simulink model "DCM_Sensing"  (R2019a)
settings: Solver=ode5  StartTime=0.0  StopTime=t_end  FixedStep=dt  RelTol=1e-3  EnableMultiTasking=on
values from neighbouring files (symbols this model uses):
  dt = 1e-5    (= 1e-05)    [Experiment_1_DCM_Parameter.m]
  dt_omega = 5e-4    (= 0.0005)    [Experiment_1_DCM_Parameter.m]
  EncoderLines = 4096    [Experiment_1_DCM_Parameter.m]
  I_AN = 1    [Experiment_1_DCM_Parameter.m]
  I_EN = 0.1    [Experiment_1_DCM_Parameter.m]
  n_Igain = 0.075    [Experiment_1_DCM_Parameter.m]
  n_Imax = 0.15    [Experiment_1_DCM_Parameter.m]
  n_Imin = -n_Imax    (= -0.15)    [Experiment_1_DCM_Parameter.m]
  T_CON = 0    [Experiment_1_DCM_Parameter.m]
  V_CON = 0    [Experiment_1_DCM_Parameter.m]
libraries: simulink x3
settings Model: Creator=BinLi  LastModifiedBy=Praktikum
settings DataIOCC: LimitDataPoints=on  SaveFormat=Array  SignalLoggingSaveFormat=ModelDataLogs  ReturnWorkspaceOutputs=off
settings OptimizationCC: ExpressionDepthLimit=2147483647  LifeSpan=inf
settings DebuggingCC: UnderspecifiedInitializationDetection=Classic  MergeDetectMultiDrivingBlocksExec=none  SolverPrmCheckMsg=warning  FcnCallInpInsideContextMsg=warning  StateNameClashWarn=warning  SFUnexpectedBacktrackingDiag=warning  SFNoUnconditionalDefaultTransitionDiag=warning  SFExecutionAtInitializationDiag=none  ArithmeticOperatorsInVariantConditions=warning
settings HardwareCC: ProdBitPerPointer=32  ProdBitPerSizeT=32  ProdBitPerPtrDiffT=32  ProdLargestAtomicFloat=None  ProdIntDivRoundTo=Undefined  ProdEndianess=Unspecified  ProdWordSize=32  ProdHWDeviceType=32-bit Generic
settings ModelReferenceCC: PropagateSignalLabelsOutOfModel=off
settings SFSimCC: SimUseLocalCustomCode=off
settings RTWCC: RTWUseLocalCustomCode=off
settings CodeAppCC: StateflowObjectComments=on
settings GRTTargetCC: TargetLangStandard=C89/C90 (ANSI)  CombineOutputUpdateFcns=off  GRTInterface=on
settings ConfigComp: CovMetricSettings=dw  CovSaveCumulativeToWorkspaceVar=on  CovSaveSingleToWorkspaceVar=on  CovExternalEMLEnable=off  CovSFcnEnable=off

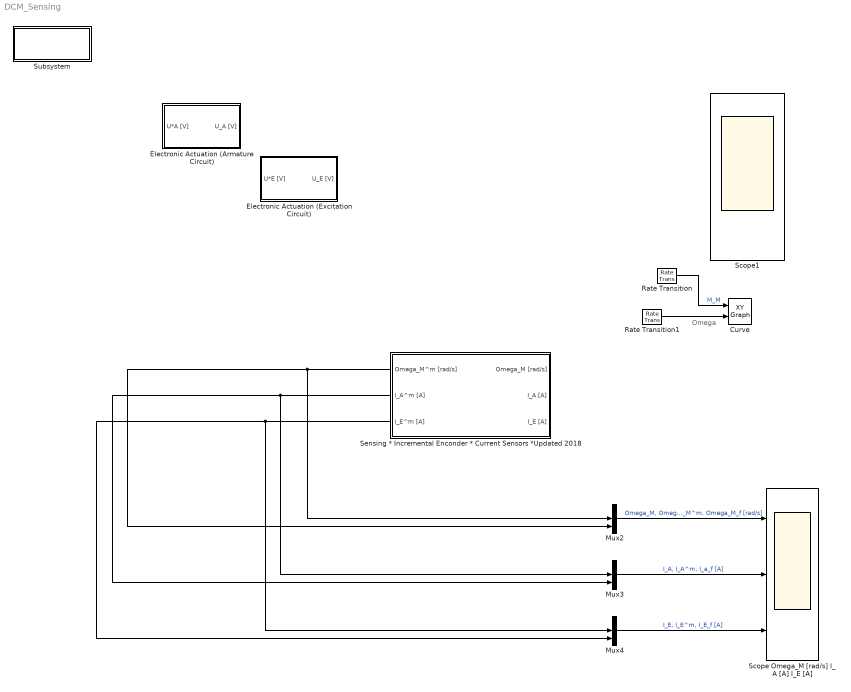
== system DCM_Sensing ==
  note: Omega
  Curve : simulink/Sinks/XY Graph  xmin=-1000  xmax=1200  ymin=-2000  ymax=2000  st=5e-3
  Electronic Actuation (Armature Circuit) : Subsystem
  Electronic Actuation (Excitation Circuit) : Subsystem
  Mux2 : Mux  Inputs=3
  Mux3 : Mux  Inputs=3
  Mux4 : Mux  Inputs=3
  Rate Transition : RateTransition
  Rate Transition1 : RateTransition
  Scope Omega_M [rad/s] I_A [A] I_E [A] : Scope  NumInputPorts=3
  Scope1 : Scope  NumInputPorts=6
  Sensing * Incremental Enconder * Current Sensors *Updated 2018 : Subsystem
  Subsystem : Subsystem
      settings: OpenFcn=Experiment_1_DCM_Parameter
      mask Display: disp('Initialize\n (doppelklicken)')
  wires:
  ? -> Scope1/1, Rate Transition1/1, Sensing * Incremental Enconder * Current Sensors *Updated 2018/1(Omega_M [rad/s]), Mux2/1  "Omega"
  ? -> Scope1/2, Sensing * Incremental Enconder * Current Sensors *Updated 2018/2(I_A [A]), Mux3/1  "I_A"
  ? -> Scope1/5, Sensing * Incremental Enconder * Current Sensors *Updated 2018/3(I_E [A]), Mux4/1  "I_E"
  ? -> Rate Transition/1, Scope1/6  "M_M"
  ? -> Scope1/3  "E_A"
  ? -> Scope1/4  "Psi_E"
  Rate Transition/1 -> Curve/1  "M_M"
  Rate Transition1/1 -> Curve/2
  Mux2/1 -> Scope Omega_M [rad/s] I_A [A] I_E [A]/1  "Omega_M, Omega_M^m, Omega_M_f [rad/s]"
  Mux3/1 -> Scope Omega_M [rad/s] I_A [A] I_E [A]/2  "I_A, I_A^m, I_a_f [A]"
  Mux4/1 -> Scope Omega_M [rad/s] I_A [A] I_E [A]/3  "I_E, I_E^m, I_E_f [A]"
  Sensing * Incremental Enconder * Current Sensors *Updated 2018/2(I_A^m [A]) -> Mux3/3, Mux3/2
  Sensing * Incremental Enconder * Current Sensors *Updated 2018/3(I_E^m [A]) -> Mux4/3, Mux4/2
  Sensing * Incremental Enconder * Current Sensors *Updated 2018/1(Omega_M^m [rad/s]) -> Mux2/3, Mux2/2

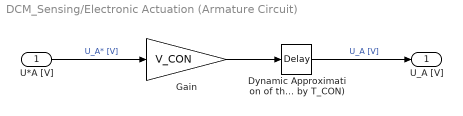
== system DCM_Sensing/Electronic Actuation (Armature Circuit) ==
  U*A [V] : Inport
  Dynamic Approximation of the 2-level-converter (Delay by T_CON) : TransportDelay  DelayTime=T_CON
  Gain : Gain  Gain=V_CON
  U_A [V] : Outport
  wires:
  Dynamic Approximation of the 2-level-converter (Delay by T_CON)/1 -> U_A [V]/1  "U_A [V]"
  U*A [V]/1 -> Gain/1  "U_A* [V]"
  Gain/1 -> Dynamic Approximation of the 2-level-converter (Delay by T_CON)/1

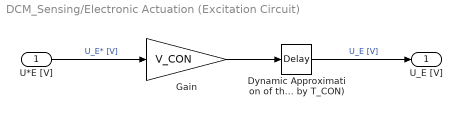
== system DCM_Sensing/Electronic Actuation (Excitation Circuit) ==
  U*E [V] : Inport
  Dynamic Approximation of the 2-level-converter (Delay by T_CON) : TransportDelay  DelayTime=T_CON
  Gain : Gain  Gain=V_CON
  U_E [V] : Outport
  wires:
  Gain/1 -> Dynamic Approximation of the 2-level-converter (Delay by T_CON)/1
  U*E [V]/1 -> Gain/1  "U_E* [V]"
  Dynamic Approximation of the 2-level-converter (Delay by T_CON)/1 -> U_E [V]/1  "U_E [V]"

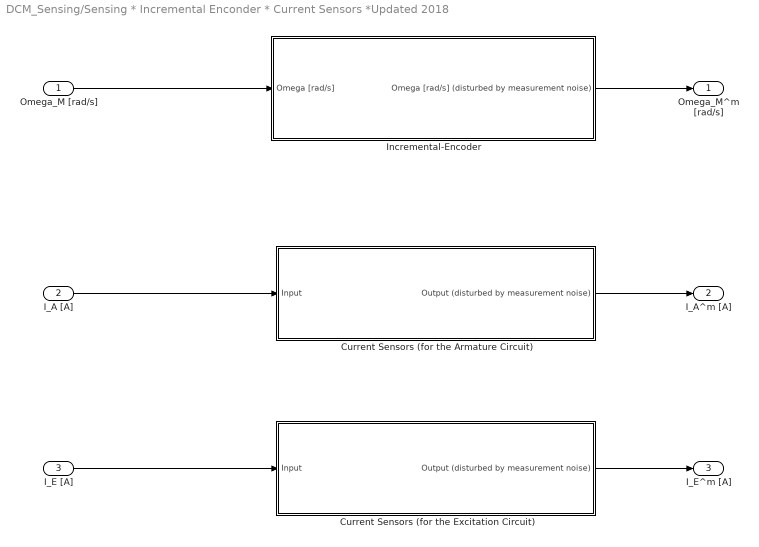
== system DCM_Sensing/Sensing * Incremental Enconder * Current Sensors *Updated 2018 ==
  Omega_M [rad/s] : Inport
  I_A [A] : Inport  Port=2
  I_E [A] : Inport  Port=3
  Current Sensors (for the Armature Circuit) : Subsystem  mask(Noise Generator){Noise_Power=0.1*dt, h_Noise=dt, V_Noise=n_Igain, Max_Noise=n_Imax*I_AN, Min_Noise=n_Imin*I_AN}
      mask prompts: Noise_Power "Noise Power (default: 0.1*h)"; h_Noise "Noise Sampling Time (default: h)"; V_Noise "Noise Gain (Amplification)"; Max_Noise "Maximal Noise Amplitude (Saturation)"; Min_Noise "Minimal Noise Amplitude (Saturation)"
      mask help:
      | This block generates sensor noise (band limited white noise) at a noise sampling time h_Noise [s, default: h] and with a noise power Noise_Power [1, default: 0.1*h], to produce normally distributed bandlimited white noise with a maximal amplitude around 1.
      | The noise amplitude can be amplified with a noise gain V_Noise [1] and saturated with the maximal and minimal noise amplitude selection.
      | With the flag "ENABLE_NOISE" (constant) the noise output can be activated or set to zero.
      mask Display:
      | fprintf('Noise Power: %1.3f [1]\n Noise Sampling Time: %1.3f [s] \n Noise Gain: %g [1] \n Saturation: [%g,%g]'...
      |    ,Noise_Power, h_Noise, V_Noise, Min_Noise, Max_Noise);
      | port_label('input',1,'I [A]');
      | port_label('output',1,'I^m [A]');
  "Current Sensors (for the Excitation Circuit) " : Subsystem  mask(Noise Generator){Noise_Power=0.1*dt, h_Noise=dt, V_Noise=n_Igain, Max_Noise=n_Imax*I_EN, Min_Noise=n_Imin*I_EN}
      mask prompts: Noise_Power "Noise Power (default: 0.1*h)"; h_Noise "Noise Sampling Time (default: h)"; V_Noise "Noise Gain (Amplification)"; Max_Noise "Maximal Noise Amplitude (Saturation)"; Min_Noise "Minimal Noise Amplitude (Saturation)"
      mask help:
      | This block generates sensor noise (band limited white noise) at a noise sampling time h_Noise [s, default: h] and with a noise power Noise_Power [1, default: 0.1*h], to produce normally distributed bandlimited white noise with a maximal amplitude around 1.
      | The noise amplitude can be amplified with a noise gain V_Noise [1] and saturated with the maximal and minimal noise amplitude selection.
      | With the flag "ENABLE_NOISE" (constant) the noise output can be activated or set to zero.
      mask Display:
      | fprintf('Noise Power: %1.3f [1]\n Noise Sampling Time: %1.3f [s] \n Noise Gain: %g [1] \n Saturation: [%g,%g]'...
      |    ,Noise_Power, h_Noise, V_Noise, Min_Noise, Max_Noise);
      | port_label('input',1,'I [A]');
      | port_label('output',1,'I^m [A]');
  Incremental-Encoder : Subsystem  mask(Noise Generator){enc_lines=EncoderLines}
      mask prompts: enc_lines "Encoder Lines"
      mask help:
      | This block generates sensor noise (band limited white noise) at a noise sampling time h_Noise [s, default: h] and with a noise power Noise_Power [1, default: 0.1*h], to produce normally distributed bandlimited white noise with a maximal amplitude around 1.
      | The noise amplitude can be amplified with a noise gain V_Noise [1] and saturated with the maximal and minimal noise amplitude selection.
      | With the flag "ENABLE_NOISE" (constant) the noise output can be activated or set to zero.
      mask Display:
      | fprintf('Encoder Lines %g [1]',enc_lines);
      | port_label('input',1,'Omega [rad/s]');
      | port_label('output',1,'Omega^m [rad/s]');
  Omega_M^m [rad/s] : Outport  InitialOutput=0
  I_A^m [A] : Outport  Port=2  InitialOutput=0
  I_E^m [A] : Outport  Port=3  InitialOutput=0
  wires:
  Omega_M [rad/s]/1 -> Incremental-Encoder/1(Omega [rad/s])
  I_A [A]/1 -> Current Sensors (for the Armature Circuit)/1(Input)
  I_E [A]/1 -> "Current Sensors (for the Excitation Circuit) "/1(Input)
  "Current Sensors (for the Excitation Circuit) "/1(Output (disturbed by measurement noise)) -> I_E^m [A]/1
  Current Sensors (for the Armature Circuit)/1(Output (disturbed by measurement noise)) -> I_A^m [A]/1
  Incremental-Encoder/1(Omega [rad/s] (disturbed by measurement noise)) -> Omega_M^m [rad/s]/1

== system DCM_Sensing/Subsystem ==

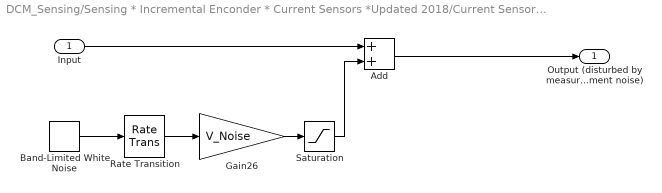
== system DCM_Sensing/Sensing * Incremental Enconder * Current Sensors *Updated 2018/Current Sensors (for the Armature Circuit) ==
  Input : Inport
  Add : Sum
  Band-Limited White Noise : simulink/Sources/Band-Limited White Noise  Cov=[Noise_Power]  Ts=h_Noise  seed=[23341]
  Gain26 : Gain  Gain=V_Noise
  Rate Transition : RateTransition  OutPortSampleTime=h_Noise
  Saturation : Saturate  UpperLimit=Max_Noise  LowerLimit=Min_Noise
  Output (disturbed by measurement noise) : Outport
  wires:
  Saturation/1 -> Add/2
  Input/1 -> Add/1
  Rate Transition/1 -> Gain26/1
  Gain26/1 -> Saturation/1
  Band-Limited White Noise/1 -> Rate Transition/1
  Add/1 -> Output (disturbed by measurement noise)/1

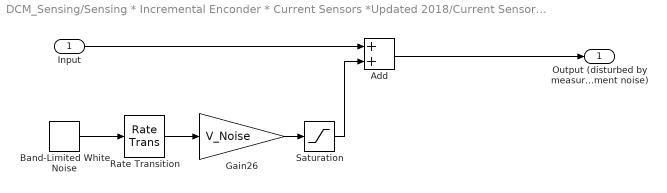
== system DCM_Sensing/Sensing * Incremental Enconder * Current Sensors *Updated 2018/Current Sensors (for the Excitation Circuit)  ==
  Input : Inport
  Add : Sum
  Band-Limited White Noise : simulink/Sources/Band-Limited White Noise  Cov=[Noise_Power]  Ts=h_Noise  seed=[23341]
  Gain26 : Gain  Gain=V_Noise
  Rate Transition : RateTransition  OutPortSampleTime=h_Noise
  Saturation : Saturate  UpperLimit=Max_Noise  LowerLimit=Min_Noise
  Output (disturbed by measurement noise) : Outport
  wires:
  Band-Limited White Noise/1 -> Rate Transition/1
  Gain26/1 -> Saturation/1
  Rate Transition/1 -> Gain26/1
  Input/1 -> Add/1
  Saturation/1 -> Add/2
  Add/1 -> Output (disturbed by measurement noise)/1

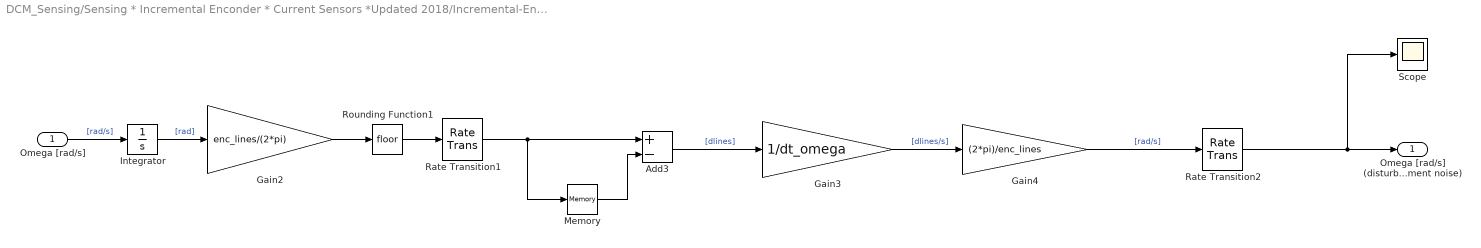
== system DCM_Sensing/Sensing * Incremental Enconder * Current Sensors *Updated 2018/Incremental-Encoder ==
  Omega [rad/s] : Inport
  Add3 : Sum  Inputs=+-
  Gain2 : Gain  Gain=enc_lines/(2*pi)
  Gain3 : Gain  Gain=1/dt_omega
  Gain4 : Gain  Gain=(2*pi)/enc_lines
  Integrator : Integrator
  Memory : Memory  InheritSampleTime=on
  Rate Transition1 : RateTransition  OutPortSampleTime=dt_omega
  Rate Transition2 : RateTransition  OutPortSampleTime=dt
  Rounding Function1 : Rounding
  Scope : Scope
  Omega [rad/s] (disturbed by measurement noise) : Outport
  wires:
  Integrator/1 -> Gain2/1  "[rad]"
  Gain2/1 -> Rounding Function1/1
  Memory/1 -> Add3/2
  Add3/1 -> Gain3/1  "[dlines]"
  Gain3/1 -> Gain4/1  "[dlines/s]"
  Gain4/1 -> Rate Transition2/1  "[rad/s]"
  Rounding Function1/1 -> Rate Transition1/1
  Omega [rad/s]/1 -> Integrator/1  "[rad/s]"
  Rate Transition1/1 -> Memory/1, Add3/1
  Rate Transition2/1 -> Omega [rad/s] (disturbed by measurement noise)/1, Scope/1
